simulink model "LandingSimulation_simple"  (R2015a)
settings: Solver=ode45  StartTime=0.0  StopTime=100  FixedStep=.1  RelTol=1e-10
values from neighbouring files (symbols this model uses):
  g0 = Planet_MU/Planet_Radius^2    (= 1.62845995)    [Constants.m]    (also in Constants_simple.m = 10)
  Starting_X_Speed = 100    [Constants_simple.m]    (also in StartingSpeed.m = V_per)
  Starting_Y_Speed = -25    [Constants_simple.m]    (also in StartingSpeed.m = 0)
  TWR = 2.5    [Constants_simple.m]    (also in SolverSuicideBurn.m = TWR_plot(j); SolverSuicideBurn_Terrain.m = TWR_plot(j))
  TWR_x = TWR*cosd(theta)    [SimpleSolver.m]    (also in SimplerSolver.m)
  TWR_y = TWR*sind(theta)    [SimpleSolver.m]    (also in SimplerSolver.m)
libraries: simulink x2, vrlib x1
settings Model: Creator=raulm_000  LastModifiedBy=raulm_000

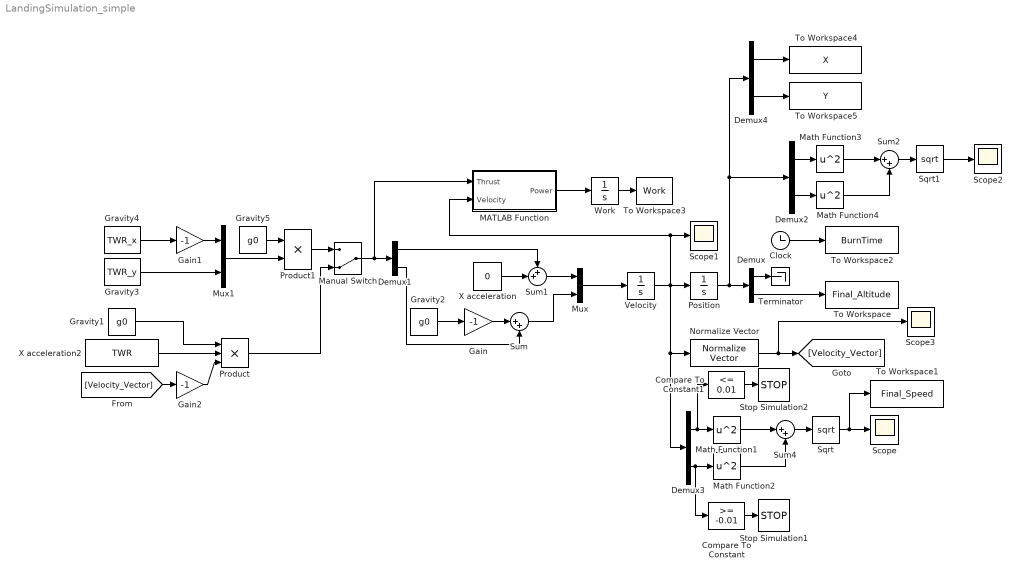
== system LandingSimulation_simple ==
  Clock : Clock
  Compare To Constant : simulink/Logic and Bit Operations/Compare To Constant  relop=>=  const=-0.01  OutDataTypeStr=boolean
  Compare To Constant1 : simulink/Logic and Bit Operations/Compare To Constant  relop=<=  const=0.01  OutDataTypeStr=boolean
  Demux{,1..4} (5 alike) : Demux  Outputs=2
  Gain : Gain  Gain=-1
  Gain1 : Gain  Gain=-1
  Gain2 : Gain  Gain=-1
  Gravity1 : Constant  Value=g0
  Gravity2 : Constant  Value=g0
  Gravity3 : Constant  Value=TWR_y
  Gravity4 : Constant  Value=TWR_x
  Gravity5 : Constant  Value=g0
  MATLAB Function : MATLAB Function  TreatAsAtomicUnit=on
  Manual Switch : ManualSwitch  CurrentSetting=0
  Math Function{1..4} (4 alike) : Math  Operator=square  SaturateOnIntegerOverflow=on
  Mux : Mux  Inputs=2
  Mux1 : Mux  Inputs=2
  Normalize Vector : vrlib/Utilities/Normalize Vector  maxzero=0
  Position : Integrator  InitialCondition=[0,0]
  Product : Product  Inputs=3
  Product1 : Product
  Scope{,1..3} (4 alike) : Scope
      Scope settings: YMin=0.00075  YMax=0.00375
      Scope1 settings: YMin=0.00075  YMax=0.00375
      Scope2 settings: YMin=0.00075  YMax=0.00375  SaveName=ScopeData2
      Scope3 settings: YMin=0.00075  YMax=0.00375  SaveName=ScopeData3
  Sqrt : Sqrt  SaturateOnIntegerOverflow=on
  Sqrt1 : Sqrt  SaturateOnIntegerOverflow=on
  Stop Simulation1 : Stop
  Stop Simulation2 : Stop
  Sum : Sum  Inputs=|++
  Sum1 : Sum  Inputs=++|
  Sum2 : Sum  Inputs=|++
  Sum4 : Sum  Inputs=|++
  Terminator : Terminator
  To Workspace : ToWorkspace  VariableName=Final_Altitude  SampleTime=-1
      settings: MaxDataPoints=1
  To Workspace1 : ToWorkspace  VariableName=Final_Speed  SampleTime=-1
      settings: MaxDataPoints=1
  To Workspace2 : ToWorkspace  VariableName=BurnTime  SampleTime=-1
      settings: MaxDataPoints=1
  To Workspace3 : ToWorkspace  VariableName=Work  SampleTime=-1
      settings: MaxDataPoints=1
  To Workspace4 : ToWorkspace  VariableName=X  SampleTime=-1
  To Workspace5 : ToWorkspace  VariableName=Y  SampleTime=-1
  Velocity : Integrator  InitialCondition=[Starting_X_Speed,Starting_Y_Speed]
  Work : Integrator
  X acceleration : Constant  Value=0
  X acceleration2 : Constant  Value=TWR
  wires:
  Mux/1 -> Velocity/1
  Gravity2/1 -> Gain/1
  Position/1 -> Demux4/1, Demux2/1, Demux/1
  Normalize Vector/1 -> Scope3/1, [Velocity_Vector]
  Gain/1 -> Sum/1
  Sum/1 -> Mux/2
  X acceleration/1 -> Sum1/2
  Sum1/1 -> Mux/1
  Velocity/1 -> Demux3/1, Normalize Vector/1, Scope1/1, MATLAB Function/2(Velocity), Position/1
  Demux1/2 -> Sum/2
  Demux3/2 -> Compare To Constant/1, Math Function2/1
  Math Function1/1 -> Sum4/1
  Math Function2/1 -> Sum4/2
  Sum4/1 -> Sqrt/1
  Sqrt/1 -> To Workspace1/1, Scope/1
  Compare To Constant/1 -> Stop Simulation1/1
  [Velocity_Vector] -> Gain2/1
  X acceleration2/1 -> Product/2
  Gain2/1 -> Product/3
  Gravity1/1 -> Product/1
  Demux3/1 -> Compare To Constant1/1, Math Function1/1
  Demux/2 -> To Workspace/1
  Demux1/1 -> Sum1/1
  Demux/1 -> Terminator/1
  Clock/1 -> To Workspace2/1
  Manual Switch/1 -> MATLAB Function/1(Thrust), Demux1/1
  Product/1 -> Manual Switch/2
  Gravity3/1 -> Mux1/2
  Gravity4/1 -> Gain1/1
  Gain1/1 -> Mux1/1
  Product1/1 -> Manual Switch/1
  Mux1/1 -> Product1/2
  Gravity5/1 -> Product1/1
  Demux2/2 -> Math Function4/1
  Demux2/1 -> Math Function3/1
  Math Function3/1 -> Sum2/1
  Math Function4/1 -> Sum2/2
  Sum2/1 -> Sqrt1/1
  Sqrt1/1 -> Scope2/1
  Compare To Constant1/1 -> Stop Simulation2/1
  MATLAB Function/1(Power) -> Work/1
  Work/1 -> To Workspace3/1
  Demux4/1 -> To Workspace4/1
  Demux4/2 -> To Workspace5/1

== matlab function LandingSimulation_simple/MATLAB Function ==
  data: Thrust input; Power output; Velocity input
function Power = fcn(Thrust,Velocity)
%#codegen

Power = dot(Thrust,Velocity);
